simulink model "Torque_Controller"  (R2024b)
settings: Solver=VariableStepAuto  StartTime=0.0  StopTime=10.0  RelTol=1e-3
settings Model: Creator=junhyeongdoh  LastModifiedBy=junhyeongdoh

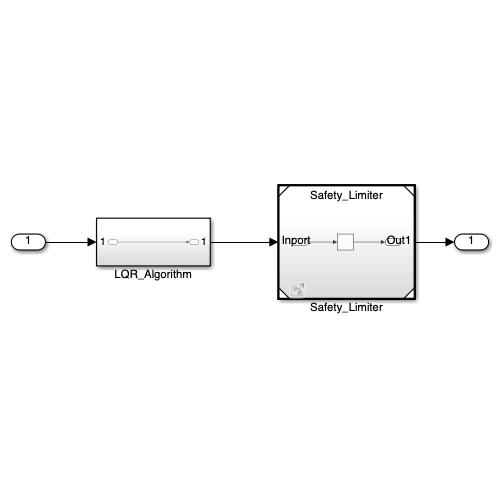
[thumbnail: Simulink's stored preview of the top-level diagram]
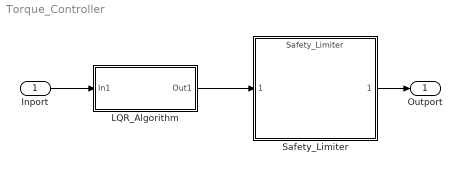
== system Torque_Controller ==
  Inport : Inport
  LQR_Algorithm : Subsystem
  Safety_Limiter : ModelReference  ModelNameDialog=Safety_Limiter.slx  SimulationMode=Normal  ModelReferenceVersion=1.1
  Outport : Outport
  wires:
  Inport/1 -> LQR_Algorithm/1(In1)
  LQR_Algorithm/1(Out1) -> Safety_Limiter/1
  Safety_Limiter/1 -> Outport/1

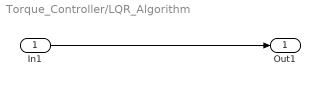
== system Torque_Controller/LQR_Algorithm ==
  In1 : Inport
  Out1 : Outport
  wires:
  In1/1 -> Out1/1
